simulink model "filterAnalyse"  (R2018a)
settings: Solver=ode4  StartTime=0.0  StopTime=simTime  FixedStep=stepTime  RelTol=1e-3
values from neighbouring files (symbols this model uses):
  minmaxBuffer = 64    [heartrate.m]
  normalizeBPMBuffer = 200    [heartrate.m]
  normalizeBufferSize = 64    [heartrate.m]
  stepTime = mean(diff(t))    [heartrate.m]    (also in heartrate_example.mat = 0.04)
libraries: dspstat3 x6, simulink x4
settings Model: Creator=Don  LastModifiedBy=Don

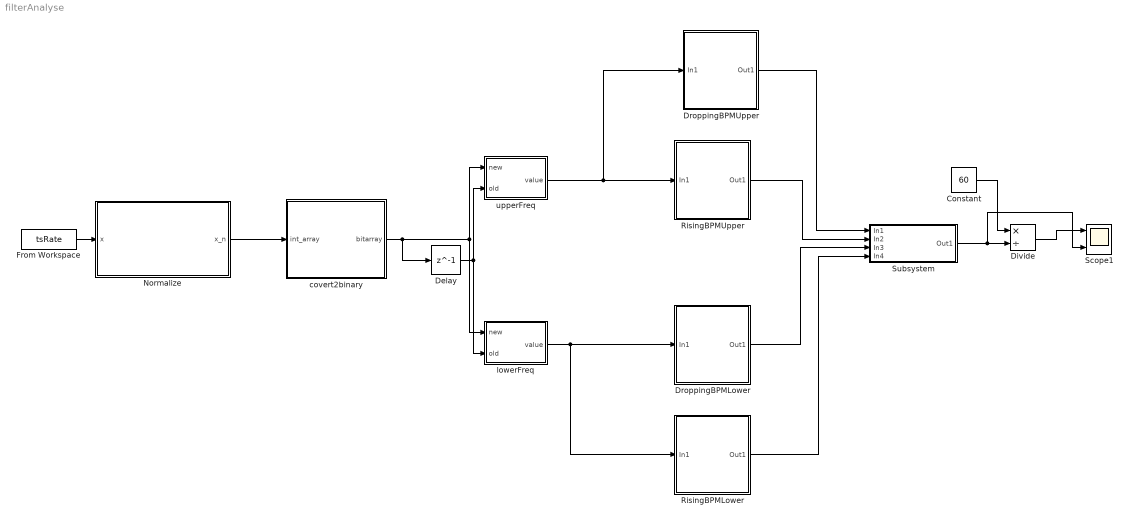
== system filterAnalyse ==
  Constant : Constant  Value=60
  Delay : Delay  DelayLength=1
  Divide : Product  Inputs=*/
  DroppingBPMLower : Subsystem
  DroppingBPMUpper : Subsystem
  From Workspace : FromWorkspace  VariableName=tsRate  SampleTime=stepTime  Interpolate=off  OutputAfterFinalValue=Setting to zero
  Normalize : Subsystem
  RisingBPMLower : Subsystem
  RisingBPMUpper : Subsystem
  Scope1 : Scope  NumInputPorts=2
  Subsystem : Subsystem
  covert2binary : Subsystem
  lowerFreq : MATLAB Function  TreatAsAtomicUnit=on
  upperFreq : MATLAB Function  TreatAsAtomicUnit=on
  wires:
  upperFreq/1(value) -> DroppingBPMUpper/1(In1), RisingBPMUpper/1(In1)
  Delay/1 -> lowerFreq/2(old), upperFreq/2(old)
  lowerFreq/1(value) -> RisingBPMLower/1(In1), DroppingBPMLower/1(In1)
  From Workspace/1 -> Normalize/1(x)
  covert2binary/1(bitarray) -> Delay/1, lowerFreq/1(new), upperFreq/1(new)
  Normalize/1(x_n) -> covert2binary/1(int_array)
  RisingBPMUpper/1(Out1) -> Subsystem/2(In2)
  DroppingBPMLower/1(Out1) -> Subsystem/3(In3)
  DroppingBPMUpper/1(Out1) -> Subsystem/1(In1)
  RisingBPMLower/1(Out1) -> Subsystem/4(In4)
  Subsystem/1(Out1) -> Divide/2, Scope1/2
  Constant/1 -> Divide/1
  Divide/1 -> Scope1/1

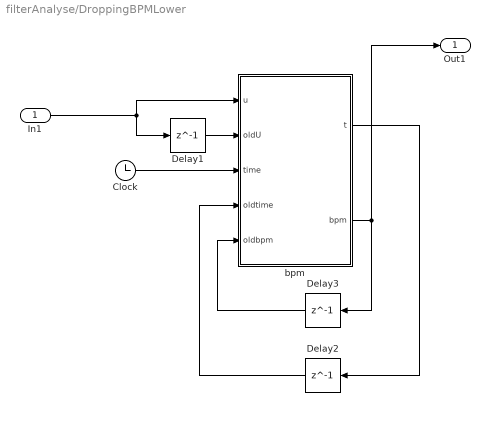
== system filterAnalyse/DroppingBPMLower ==
  In1 : Inport
  Clock : Clock
  Delay1 : Delay  DelayLength=1
  Delay2 : Delay  DelayLength=1
  Delay3 : Delay  DelayLength=1
  "bpm " : MATLAB Function  TreatAsAtomicUnit=on
  Out1 : Outport
  wires:
  Delay1/1 -> "bpm "/2(oldU)
  In1/1 -> Delay1/1, "bpm "/1(u)
  "bpm "/2(bpm) -> Out1/1, Delay3/1
  "bpm "/1(t) -> Delay2/1
  Delay2/1 -> "bpm "/4(oldtime)
  Delay3/1 -> "bpm "/5(oldbpm)
  Clock/1 -> "bpm "/3(time)

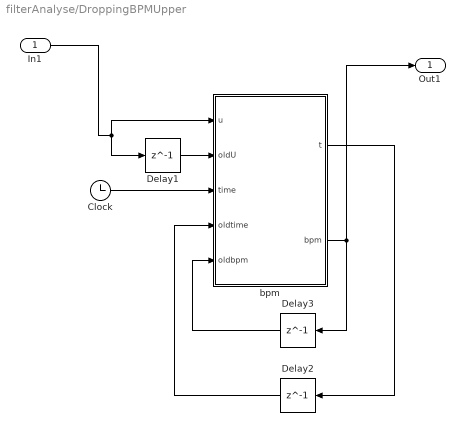
== system filterAnalyse/DroppingBPMUpper ==
  In1 : Inport
  Clock : Clock
  Delay1 : Delay  DelayLength=1
  Delay2 : Delay  DelayLength=1
  Delay3 : Delay  DelayLength=1
  "bpm " : MATLAB Function  TreatAsAtomicUnit=on
  Out1 : Outport
  wires:
  Delay1/1 -> "bpm "/2(oldU)
  In1/1 -> Delay1/1, "bpm "/1(u)
  "bpm "/2(bpm) -> Out1/1, Delay3/1
  "bpm "/1(t) -> Delay2/1
  Delay2/1 -> "bpm "/4(oldtime)
  Delay3/1 -> "bpm "/5(oldbpm)
  Clock/1 -> "bpm "/3(time)

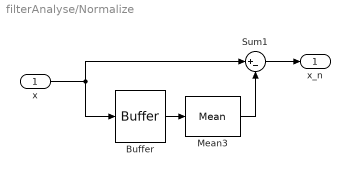
== system filterAnalyse/Normalize ==
  x : Inport
  Buffer : Buffer  N=normalizeBufferSize  OutputFrames=off
  Mean3 : dspstat3/Mean  run=off  InputProcessing=Columns as channels (frame based)  reset_popup=None  directionMode=Each column  dimension=1  roiEnable=off  roiType=Rectangles  roiPortion=Entire ROI  roiOutput=Individual statistics for each ROI  roiFlag=off  roundingMode=Floor  overflowMode=off  outputDataTypeStr=Inherit: Same as accumulator  outputMin=[]  outputMax=[]  outputLastDataTypeStr=Inherit: Same as accumulator
  Sum1 : Sum  Inputs=|+-
  x_n : Outport
  wires:
  Mean3/1 -> Sum1/2
  Buffer/1 -> Mean3/1
  Sum1/1 -> x_n/1
  x/1 -> Buffer/1, Sum1/1

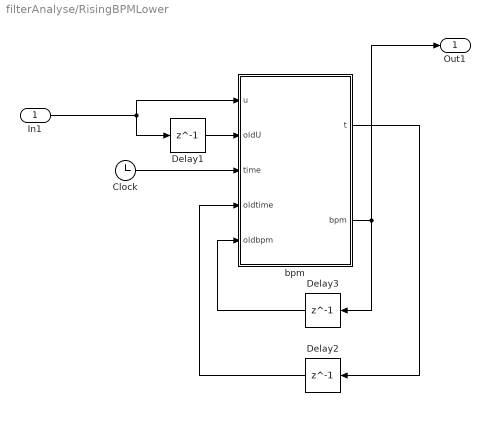
== system filterAnalyse/RisingBPMLower ==
  In1 : Inport
  Clock : Clock
  Delay1 : Delay  DelayLength=1
  Delay2 : Delay  DelayLength=1
  Delay3 : Delay  DelayLength=1
  "bpm " : MATLAB Function  TreatAsAtomicUnit=on
  Out1 : Outport
  wires:
  Clock/1 -> "bpm "/3(time)
  Delay3/1 -> "bpm "/5(oldbpm)
  Delay2/1 -> "bpm "/4(oldtime)
  "bpm "/1(t) -> Delay2/1
  "bpm "/2(bpm) -> Delay3/1, Out1/1
  In1/1 -> "bpm "/1(u), Delay1/1
  Delay1/1 -> "bpm "/2(oldU)

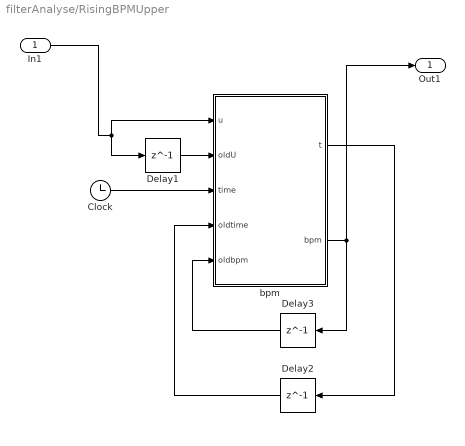
== system filterAnalyse/RisingBPMUpper ==
  In1 : Inport
  Clock : Clock
  Delay1 : Delay  DelayLength=1
  Delay2 : Delay  DelayLength=1
  Delay3 : Delay  DelayLength=1
  "bpm " : MATLAB Function  TreatAsAtomicUnit=on
  Out1 : Outport
  wires:
  Delay1/1 -> "bpm "/2(oldU)
  In1/1 -> Delay1/1, "bpm "/1(u)
  "bpm "/2(bpm) -> Out1/1, Delay3/1
  "bpm "/1(t) -> Delay2/1
  Delay2/1 -> "bpm "/4(oldtime)
  Delay3/1 -> "bpm "/5(oldbpm)
  Clock/1 -> "bpm "/3(time)

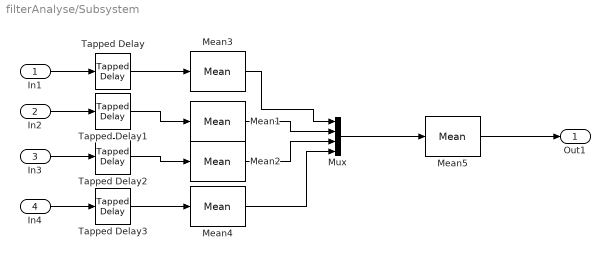
== system filterAnalyse/Subsystem ==
  In1 : Inport
  In2 : Inport  Port=2
  In3 : Inport  Port=3
  In4 : Inport  Port=4
  Mean{1..5} (5 alike) : dspstat3/Mean  run=off  InputProcessing=Columns as channels (frame based)  reset_popup=None  directionMode=Each column  dimension=1  roiEnable=off  roiType=Rectangles  roiPortion=Entire ROI  roiOutput=Individual statistics for each ROI  roiFlag=off  roundingMode=Floor  overflowMode=off  outputDataTypeStr=Inherit: Same as accumulator  outputMin=[]  outputMax=[]  outputLastDataTypeStr=Inherit: Same as accumulator
  Mux : Mux
  Tapped Delay{,1..3} (4 alike) : simulink/Discrete/Tapped Delay  vinit=0.0  samptime=-1  NumDelays=normalizeBPMBuffer  DelayOrder=Oldest  includeCurrent=off
  Out1 : Outport
  wires:
  In1/1 -> Tapped Delay/1
  In2/1 -> Tapped Delay1/1
  In4/1 -> Tapped Delay3/1
  In3/1 -> Tapped Delay2/1
  Tapped Delay/1 -> Mean3/1
  Tapped Delay1/1 -> Mean1/1
  Tapped Delay2/1 -> Mean2/1
  Tapped Delay3/1 -> Mean4/1
  Mean2/1 -> Mux/3
  Mean4/1 -> Mux/4
  Mean1/1 -> Mux/2
  Mean3/1 -> Mux/1
  Mux/1 -> Mean5/1
  Mean5/1 -> Out1/1

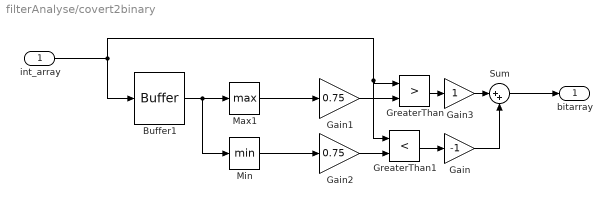
== system filterAnalyse/covert2binary ==
  int_array : Inport
  Buffer1 : Buffer  N=minmaxBuffer  OutputFrames=off
  Gain : Gain  Gain=-1
  Gain1 : Gain  Gain=0.75
  Gain2 : Gain  Gain=0.75
  Gain3 : Gain
  GreaterThan : RelationalOperator  Operator=>  OutDataTypeStr=boolean  RndMeth=Simplest
  GreaterThan1 : RelationalOperator  Operator=<  OutDataTypeStr=boolean  RndMeth=Simplest
  Max1 : MinMax  Function=max
  Min : MinMax
  Sum : Sum  Inputs=|++
  bitarray : Outport
  wires:
  int_array/1 -> Buffer1/1, GreaterThan/1, GreaterThan1/1
  Gain2/1 -> GreaterThan1/2
  Sum/1 -> bitarray/1
  Max1/1 -> Gain1/1
  Gain3/1 -> Sum/1
  Min/1 -> Gain2/1
  Buffer1/1 -> Min/1, Max1/1
  Gain/1 -> Sum/2
  GreaterThan1/1 -> Gain/1
  Gain1/1 -> GreaterThan/2
  GreaterThan/1 -> Gain3/1

== matlab function filterAnalyse/lowerFreq ==
  data: new input; value output; old input
function value = fcn(new, old)
    value = 0;
    if(new == 0)
        if(old == -1)
            value = 1;
        end
    end
   
end

== matlab function filterAnalyse/upperFreq ==
  data: new input; value output; old input
function value = fcn(new, old)
    value = 0;
    if(new == 1)
        if(old == 0)
            value = 1;
        end
    end
   
end

== matlab function filterAnalyse/RisingBPMUpper/bpm  ==
  data: u input; oldU input; t output; time input; oldtime input; bpm output; oldbpm input
function [t, bpm] = fcn(u, oldU, time, oldtime, oldbpm)
        t = oldtime;
        bpm = oldbpm;
        if(oldU == 0)
            if(u == 1)
                t = time;
                bpm = time - oldtime;
            end
        end
end

== matlab function filterAnalyse/DroppingBPMLower/bpm  ==
  data: u input; oldU input; t output; time input; oldtime input; bpm output; oldbpm input
function [t, bpm] = fcn(u, oldU, time, oldtime, oldbpm)
        t = oldtime;
        bpm = oldbpm;
        if(oldU == 0)
            if(u == 1)
                t = time;
                bpm = time - oldtime;
            end
        end
end

== matlab function filterAnalyse/RisingBPMLower/bpm  ==
  data: u input; oldU input; t output; time input; oldtime input; bpm output; oldbpm input
function [t, bpm] = fcn(u, oldU, time, oldtime, oldbpm)
        t = oldtime;
        bpm = oldbpm;
        if(oldU == 1)
            if(u == 0)
                t = time;
                bpm = time - oldtime;
            end
        end
end

== matlab function filterAnalyse/DroppingBPMUpper/bpm  ==
  data: u input; oldU input; t output; time input; oldtime input; bpm output; oldbpm input
function [t, bpm] = fcn(u, oldU, time, oldtime, oldbpm)
        t = oldtime;
        bpm = oldbpm;
        if(oldU == 1)
            if(u == 0)
                t = time;
                bpm = time - oldtime;
            end
        end
end
